simulink library "component_lib"  (R2020b)
settings: Solver=VariableStepAuto  StartTime=0.0  StopTime=10.0  RelTol=1e-3
undefined symbols (not defined in the file or in its folder): ECCV_r, par
libraries: base_lib x70, $bdroot x59, simulink x3, pid_lib x1
(part 1 of 3)
settings Model: Creator=maxjo65  LastModifiedBy=Max

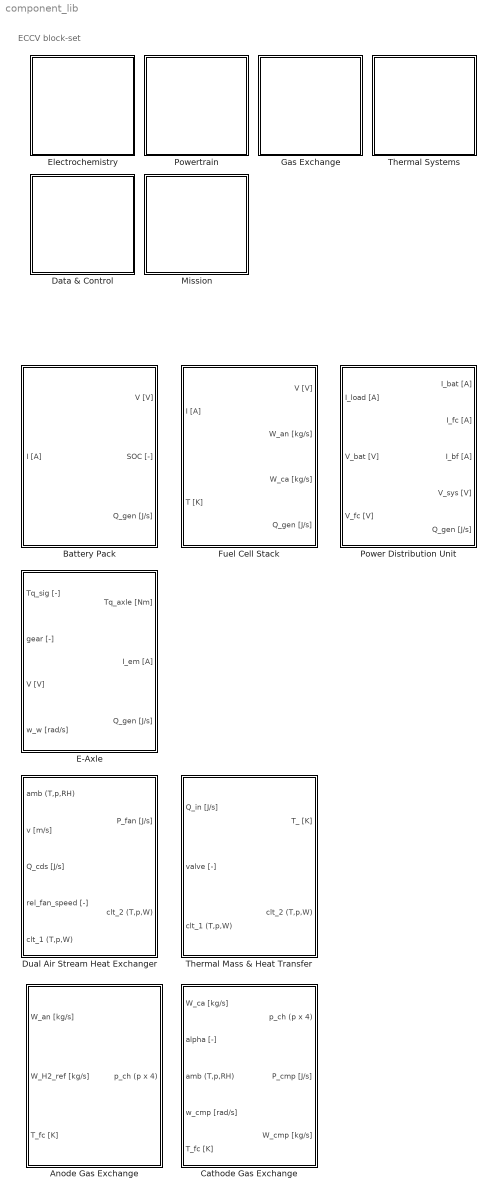
== system component_lib ==
  note: ECCV block-set
  Anode Gas Exchange : Subsystem
  Battery Pack : Subsystem  mask{SOC_0=0.5, Nx=74, Ny=6*16, T_bat=273 + 20}
      mask prompts: SOC_0 "Initial charge [-]:"; Nx "Cells in parallel  [-]:"; Ny "Cells in series [-]:"; T_bat "Temperature [K]:"
      mask init:
      | % parameter struct
      | par = struct;
      | 
      | % Get user-defined parameters
      | par.Ny = eval(get_param(gcb, 'Ny'));
      | par.Nx = eval(get_param(gcb, 'Nx'));
  Cathode Gas Exchange : Subsystem  mask{n_cell=335}
      mask prompts: n_cell "Nr. of cells [-]:"
  Data & Control : Subsystem
  Dual Air Stream Heat Exchanger : Subsystem  mask{HtH=1.1, StS=0.95}
      mask prompts: HtH "Header to header [m]"; StS "Sideplate to sideplate [m]"
  E-Axle : Subsystem  mask{n=2}
      mask prompts: n "Nr. of motors [-]"
  Electrochemistry : Subsystem
  Fuel Cell Stack : Subsystem  mask{N_series=335}
      mask prompts: N_series "Cells in series [#]:"
      mask init:
      | % parameter struct
      | par = struct;
      | 
      | % Get user-defined parameters
      | par.N_series   = eval(get_param(gcb, 'N_series'));
  Gas Exchange : Subsystem
  Mission : Subsystem
  Power Distribution Unit : Subsystem  mask{V_sys=420, P_fc=100e3, I_bt_max=300, I_bt_min=-150, T_s=1}
      mask prompts: V_sys "System voltage [V]:"; P_fc "Fuel cell power reference [J/s]:"; I_bt_max "Max. Battery current [A]"; I_bt_min "Min. Battery current [A]"; T_s "F.C Dynamic load time constant [s]:"
  Powertrain : Subsystem
  Thermal Mass & Heat Transfer : Subsystem  mask{n=5, d=2e-3, L=50e-2, m=150, cp=420, T_0=273 + 20}
      mask prompts: n "Channels [-]:"; d "Hydraulic diameter [m]:"; L "Length [m]:"; m "Mass [kg]:"; cp "Heat capacity [J/kgK]:"; T_0 "Initial temperature [K]:"
  Thermal Systems : Subsystem

== system component_lib/Anode Gas Exchange ==
  W_an [kg/s] : Inport
  W_H2_ref [kg/s] : Inport  Port=2
  T_fc [K] : Inport  Port=3
  Ejector : $bdroot/Gas Exchange/GE0013_simpleEjector  C_d=1  D_t=1.84e-3  Pi_lin=0.97  c_0=0.78406  c_1=-0.85801
  GE0007_hydrogenTank : $bdroot/Gas Exchange/GE0007_hydrogenTank  V=200e-3  T_tank=300  p_out=1.2e5  init_SOC=0.9  m0=5
  GE0008_gasProperties : $bdroot/Gas Exchange/GE0008_gasProperties  SystemSampleTime=-1  VariantActivationTime=update diagram  Latency=0  AutoFrameSizeCalculation=off
  Primary manifold : $bdroot/Gas Exchange/GE0009_controlVolume  V=10e-3  p0=5e5  x0_H2=1  x0_O2=0  T0=320  RH0=0
  SC0002_signalRead1 : $bdroot/Data & Control/SC0002_signalRead  SigName=anodeSupplyPartialPressure
  SC0002_signalRead2 : $bdroot/Data & Control/SC0002_signalRead  SigName=anodeSupplyPressure
  SC0002_signalRead3 : $bdroot/Data & Control/SC0002_signalRead  SigName=anodePrimaryPartialPressure
  SC0002_signalRead4 : $bdroot/Data & Control/SC0002_signalRead  SigName=entrainment
  SC0002_signalRead5 : $bdroot/Data & Control/SC0002_signalRead  SigName=recirculation
  SC0002_signalRead6 : $bdroot/Data & Control/SC0002_signalRead  SigName=anodePrimaryPressure
  SC0002_signalRead9 : $bdroot/Data & Control/SC0002_signalRead  SigName=anodeSupplyHumidity
  Sum1 : Sum  Inputs=++|
  Sum5 : Sum  Inputs=1
  Sum8 : Sum  Inputs=-+|
  Supply Manifold : $bdroot/Gas Exchange/GE0009_controlVolume  V=40e-3  p0=1.2e5  x0_H2=1  x0_O2=0  T0=320  RH0=0
  p_ch (p x 4) : Outport
  wires:
  Supply Manifold/2 -> GE0008_gasProperties/2
  GE0008_gasProperties/1 -> SC0002_signalRead2/1
  GE0008_gasProperties/2 -> SC0002_signalRead9/1
  Primary manifold/1 -> Ejector/1, Sum5/1, SC0002_signalRead3/1
  Sum5/1 -> SC0002_signalRead6/1
  W_H2_ref [kg/s]/1 -> GE0007_hydrogenTank/1
  GE0007_hydrogenTank/1 -> Sum8/2
  Sum8/1 -> Primary manifold/1
  GE0007_hydrogenTank/2 -> Primary manifold/2
  Primary manifold/2 -> Ejector/2
  Ejector/3 -> SC0002_signalRead5/1
  Ejector/4 -> SC0002_signalRead4/1
  Supply Manifold/1 -> Ejector/3, Ejector/5, GE0008_gasProperties/1, SC0002_signalRead1/1, p_ch (p x 4)/1
  T_fc [K]/1 -> Supply Manifold/2, Ejector/4
  Ejector/1 -> Sum1/2, Sum8/1
  Sum1/1 -> Supply Manifold/1
  W_an [kg/s]/1 -> Sum1/1

== system component_lib/Battery Pack ==
  I [A] : Inport
  Cell current : $bdroot/Data & Control/SC0002_signalRead  SigName=batteryCellCurrent
  Cell voltage : $bdroot/Data & Control/SC0002_signalRead  SigName=batteryCellVoltage
  Constant1 : Constant  Value=Nx
  Constant2 : Constant  Value=Ny
  Constant3 : Constant  Value=T_bat
  Constant4 : Constant  Value=Ny
  Constant5 : Constant  Value=Nx
  Divide : Product  Inputs=*/
  EL0001_panasonicNCR18650PF : $bdroot/Electrochemistry/EL0001_panasonicNCR18650PF  init_SOC=SOC_0
  Module current : $bdroot/Data & Control/SC0002_signalRead  SigName=batteryCurrent
  Module voltage : $bdroot/Data & Control/SC0002_signalRead  SigName=batteryVoltage
  Product1 : Product
  Product2 : Product  Inputs=3
  SOC : $bdroot/Data & Control/SC0002_signalRead  SigName=stateOfCharge
  battery power loss : $bdroot/Data & Control/SC0002_signalRead  SigName=batteryPowerLoss
  cell power loss : $bdroot/Data & Control/SC0002_signalRead  SigName=batteryCellPowerLoss
  V [V] : Outport
  SOC [-] : Outport  Port=2
  Q_gen [J/s] : Outport  Port=3
  wires:
  Product1/1 -> Module voltage/1, V [V]/1
  EL0001_panasonicNCR18650PF/2 -> SOC/1, SOC [-]/1
  Constant2/1 -> Product1/1
  EL0001_panasonicNCR18650PF/1 -> Cell voltage/1, Product1/2
  Divide/1 -> EL0001_panasonicNCR18650PF/1, Cell current/1
  I [A]/1 -> Module current/1, Divide/1
  Constant1/1 -> Divide/2
  Constant3/1 -> EL0001_panasonicNCR18650PF/2
  EL0001_panasonicNCR18650PF/3 -> Q_gen [J/s]/1, Product2/1, cell power loss/1
  Constant5/1 -> Product2/3
  Constant4/1 -> Product2/2
  Product2/1 -> battery power loss/1

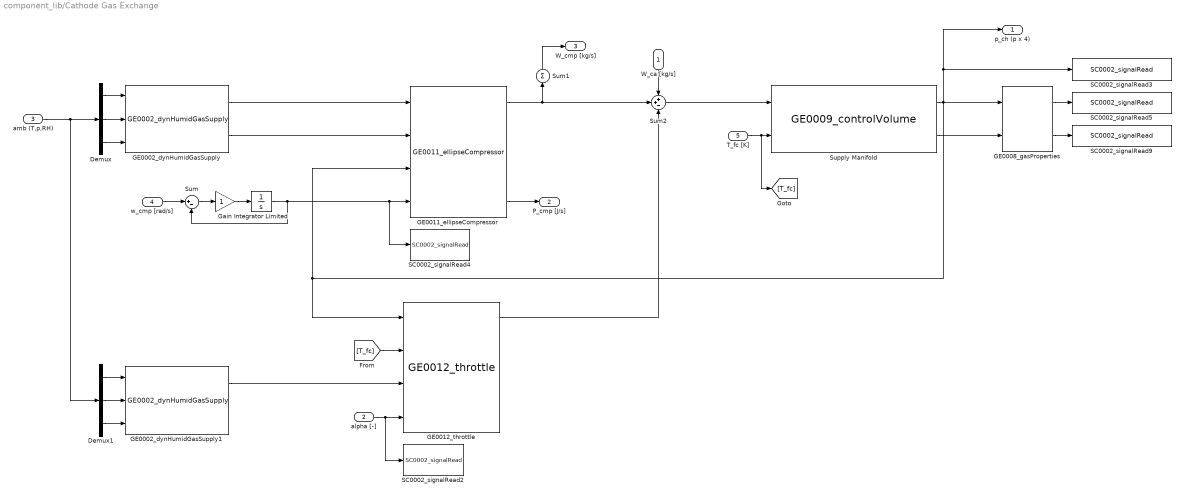
== system component_lib/Cathode Gas Exchange ==
  W_ca [kg/s] : Inport
  alpha [-] : Inport  Port=2
  amb (T,p,RH) : Inport  Port=3
  w_cmp [rad/s] : Inport  Port=4
  T_fc [K] : Inport  Port=5
  Demux : Demux  Outputs=3
  Demux1 : Demux  Outputs=3
  GE0002_dynHumidGasSupply : $bdroot/Gas Exchange/GE0002_dynHumidGasSupply  x_H2_dry=0  x_O2_dry=0.21
  GE0002_dynHumidGasSupply1 : $bdroot/Gas Exchange/GE0002_dynHumidGasSupply  x_H2_dry=0  x_O2_dry=0.21
  GE0008_gasProperties : $bdroot/Gas Exchange/GE0008_gasProperties  SystemSampleTime=-1  VariantActivationTime=update diagram  Latency=0  AutoFrameSizeCalculation=off
  GE0011_ellipseCompressor : $bdroot/Gas Exchange/GE0011_ellipseCompressor  w0=3e3
  GE0012_throttle : $bdroot/Gas Exchange/GE0012_throttle  a0=1.3229e-5  a1=9.4736e-5  a2=0.0029  Pi_lin=0.97  tan_par=1
  Gain : Gain
  Integrator Limited : Integrator  InitialCondition=1e4  LimitOutput=on  UpperSaturationLimit=2e4  LowerSaturationLimit=3e3
  SC0002_signalRead2 : $bdroot/Data & Control/SC0002_signalRead  SigName=throttlePosition
  SC0002_signalRead3 : $bdroot/Data & Control/SC0002_signalRead  SigName=cathodePartialPressure
  SC0002_signalRead4 : $bdroot/Data & Control/SC0002_signalRead  SigName=compressorSpeed
  SC0002_signalRead5 : $bdroot/Data & Control/SC0002_signalRead  SigName=cathodePressure
  SC0002_signalRead9 : $bdroot/Data & Control/SC0002_signalRead  SigName=cathodeHumidity
  Sum : Sum  Inputs=|+-
  Sum1 : Sum  Inputs=1
  Sum2 : Sum  Inputs=++-
  Supply Manifold : $bdroot/Gas Exchange/GE0009_controlVolume  V=20e-3  p0=2e5  x0_H2=0  x0_O2=0.21  T0=320  RH0=0
  p_ch (p x 4) : Outport
  P_cmp [J/s] : Outport  Port=2
  W_cmp [kg/s] : Outport  Port=3
  wires:
  GE0008_gasProperties/2 -> SC0002_signalRead9/1
  Supply Manifold/1 -> p_ch (p x 4)/1, SC0002_signalRead3/1, GE0008_gasProperties/1, GE0012_throttle/1, GE0011_ellipseCompressor/3
  GE0008_gasProperties/1 -> SC0002_signalRead5/1
  amb (T,p,RH)/1 -> Demux/1, Demux1/1
  Demux1/3 -> GE0002_dynHumidGasSupply1/3
  Demux1/2 -> GE0002_dynHumidGasSupply1/2
  Demux1/1 -> GE0002_dynHumidGasSupply1/1
  Demux/3 -> GE0002_dynHumidGasSupply/3
  Demux/2 -> GE0002_dynHumidGasSupply/2
  Demux/1 -> GE0002_dynHumidGasSupply/1
  alpha [-]/1 -> SC0002_signalRead2/1, GE0012_throttle/4
  GE0011_ellipseCompressor/4 -> P_cmp [J/s]/1
  Sum1/1 -> W_cmp [kg/s]/1
  Sum2/1 -> Supply Manifold/1
  GE0011_ellipseCompressor/1 -> Sum2/2, Sum1/1
  GE0002_dynHumidGasSupply/2 -> GE0011_ellipseCompressor/2
  T_fc [K]/1 -> [T_fc], Supply Manifold/2
  GE0002_dynHumidGasSupply1/1 -> GE0012_throttle/3
  GE0002_dynHumidGasSupply/1 -> GE0011_ellipseCompressor/1
  Supply Manifold/2 -> GE0008_gasProperties/2
  W_ca [kg/s]/1 -> Sum2/1
  GE0012_throttle/1 -> Sum2/3
  [T_fc] -> GE0012_throttle/2
  w_cmp [rad/s]/1 -> Sum/1
  Sum/1 -> Gain/1
  Integrator Limited/1 -> Sum/2, SC0002_signalRead4/1, GE0011_ellipseCompressor/4
  Gain/1 -> Integrator Limited/1

== system component_lib/Data & Control ==
  DC0006_powerSplit : Subsystem  mask{P_fc=100e3, P_fc_max=180e3, P_fc_min=10e3, T_s=1, I_bt_max=300, I_bt_min=-150}
      mask prompts: P_fc "FC power setpoint [J/s]:"; P_fc_max "Max. FC power [J/s]:"; P_fc_min "Min. FC power [J/s]:"; T_s "FC Dynamic load time constant [s]:"; I_bt_max "Max. battery current [A]:"; I_bt_min "Min. battery current [A]:"
  DC0007_cathodeFlowControl : Subsystem  mask{lambda_O2_ref=2, n_cell=455}
      mask prompts: lambda_O2_ref "Oxygen stoich. reference [-]:"; n_cell "Nr. of cells [-]:"
  DC0010_anodeTankFlowControl : Subsystem  mask{n_cell=455}
      mask prompts: n_cell "Nr. of cells [-]"
  SC0002_signalRead : Subsystem  mask{SigName=SigIdentifier}
      mask prompts: SigName "Signal identifier:"
      mask init:
      | % set name of input port
      | blockNames = Simulink.findBlocks(gcb);
      | set(blockNames(1), 'Name', SigName);
      | 
      | % log input port
      | ph = get_param([gcb, '/', SigName], 'PortHandles');
      | set_param(ph.Outport(1), 'DataLogging', 'on')
      | 
      | % set signal name in goto tag
      | set_param([gcb, '/', 'Goto'], 'GotoTag', SigName)
      mask Display: disp(SigName)
  SC0003_signalWrite : Subsystem  mask{SigName=SigIdentifier}
      mask prompts: SigName "Signal identifier:"
      mask init:
      | % set signal name in goto tag
      | set_param([gcb, '/', 'From'], 'GotoTag', SigName)
      mask Display: disp(SigName)

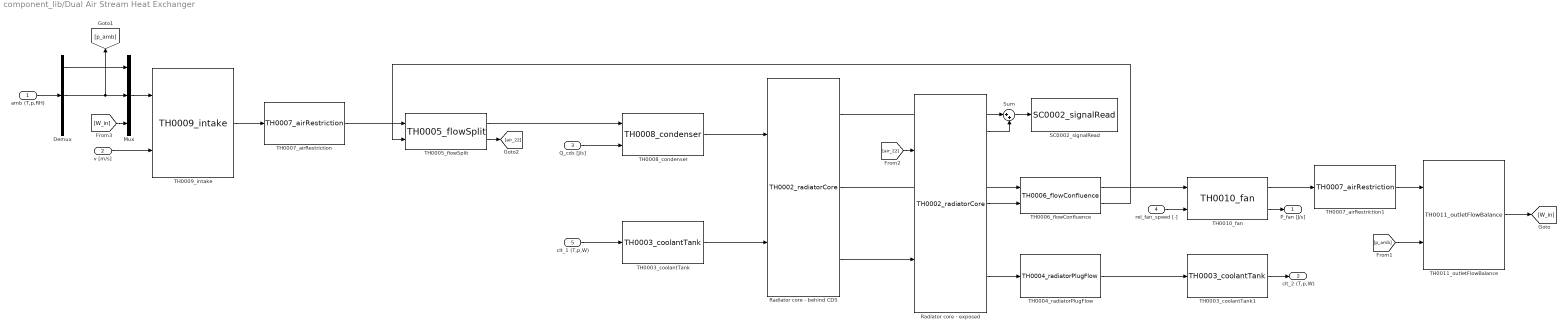
== system component_lib/Dual Air Stream Heat Exchanger ==
  amb (T,p,RH) : Inport
  v [m/s] : Inport  Port=2
  Q_cds [J/s] : Inport  Port=3
  rel_fan_speed [-] : Inport  Port=4
  clt_1 (T,p,W) : Inport  Port=5
  Demux : Demux  Outputs=3
  Mux : Mux  Inputs=3
  Radiator core - behind CDS : $bdroot/Thermal Systems/TH0002_radiatorCore  HtH=0.35  StS=0.95  radmodel=52 mm
  Radiator core - exposed : $bdroot/Thermal Systems/TH0002_radiatorCore  HtH=1.1-0.35  StS=0.95  radmodel=52 mm
  SC0002_signalRead : $bdroot/Data & Control/SC0002_signalRead  SigName=hexCoolingLoad
  Sum : Sum  Inputs=|++
  TH0003_coolantTank : $bdroot/Thermal Systems/TH0003_coolantTank  StS=0.95  D_con=0.055  T_0=286  radmodel=52 mm
  TH0003_coolantTank1 : $bdroot/Thermal Systems/TH0003_coolantTank  StS=0.95  D_con=0.055  T_0=286  radmodel=52 mm
  TH0004_radiatorPlugFlow : $bdroot/Thermal Systems/TH0004_radiatorPlugFlow  HtH=1.1  StS=0.95  T_0=286  radmodel=52 mm
  TH0005_flowSplit : $bdroot/Thermal Systems/TH0005_flowSplit  SystemSampleTime=-1  VariantActivationTime=update diagram  Latency=0  AutoFrameSizeCalculation=off
  TH0006_flowConfluence : $bdroot/Thermal Systems/TH0006_flowConfluence  gain=0.01
  TH0007_airRestriction : $bdroot/Thermal Systems/TH0007_airRestriction  A=0.8  zeta=0.3
  TH0007_airRestriction1 : $bdroot/Thermal Systems/TH0007_airRestriction  A=1  zeta=2.5
  TH0008_condenser : $bdroot/Thermal Systems/TH0008_condenser  HtH=0.85  StS=0.35  cdsmodel=18.8 mm
  TH0009_intake : $bdroot/Thermal Systems/TH0009_intake  zeta=0.9
  TH0010_fan : $bdroot/Thermal Systems/TH0010_fan  n_fan=4
  TH0011_outletFlowBalance : $bdroot/Thermal Systems/TH0011_outletFlowBalance  gain=0.05
  P_fan [J/s] : Outport
  clt_2 (T,p,W) : Outport  Port=2
  wires:
  Demux/2 -> Mux/2, [p_amb]
  Demux/1 -> Mux/1
  amb (T,p,RH)/1 -> Demux/1
  TH0003_coolantTank1/1 -> clt_2 (T,p,W)/1
  Sum/1 -> SC0002_signalRead/1
  TH0010_fan/2 -> P_fan [J/s]/1
  rel_fan_speed [-]/1 -> TH0010_fan/2
  TH0005_flowSplit/1 -> TH0008_condenser/1
  Radiator core - behind CDS/1 -> Sum/1
  v [m/s]/1 -> TH0009_intake/2
  TH0007_airRestriction/1 -> TH0005_flowSplit/1
  TH0004_radiatorPlugFlow/1 -> TH0003_coolantTank1/1
  TH0007_airRestriction1/1 -> TH0011_outletFlowBalance/1
  TH0003_coolantTank/1 -> Radiator core - behind CDS/2
  Q_cds [J/s]/1 -> TH0008_condenser/2
  clt_1 (T,p,W)/1 -> TH0003_coolantTank/1
  TH0006_flowConfluence/2 -> TH0005_flowSplit/2
  TH0006_flowConfluence/1 -> TH0010_fan/1
  Mux/1 -> TH0009_intake/1
  TH0005_flowSplit/2 -> [air_22]
  TH0009_intake/1 -> TH0007_airRestriction/1
  TH0008_condenser/1 -> Radiator core - behind CDS/1
  Radiator core - behind CDS/2 -> TH0006_flowConfluence/1
  Radiator core - exposed/2 -> TH0006_flowConfluence/2
  Radiator core - behind CDS/3 -> Radiator core - exposed/2
  [p_amb] -> TH0011_outletFlowBalance/2
  [air_22] -> Radiator core - exposed/1
  TH0010_fan/1 -> TH0007_airRestriction1/1
  Radiator core - exposed/3 -> TH0004_radiatorPlugFlow/1
  TH0011_outletFlowBalance/1 -> [W_in]
  Radiator core - exposed/1 -> Sum/2
  [W_in] -> Mux/3

== system component_lib/E-Axle ==
  note: Input as % of max. torque at current speed
  Tq_sig [-] : Inport
  gear [-] : Inport  Port=2
  V [V] : Inport  Port=3
  w_w [rad/s] : Inport  Port=4
  Constant3 : Constant
  Current sensor : $bdroot/Data & Control/SC0002_signalRead  SigName=motorCurrent
  Divide3 : Product  Inputs=**
  Gain : Gain  Gain=n
  Gain1 : Gain  Gain=n
  Gain2 : Gain  Gain=n
  Max torque : $bdroot/Data & Control/SC0002_signalRead  SigName=maxMotorTorque
  PT0002_simpleMotor : $bdroot/Powertrain/PT0002_simpleMotor  T_s=0.1
  PT0003_gearBox : $bdroot/Powertrain/PT0003_gearBox  fd_ratio=5  gear_ratios=[1, 1]  eta_gb=0.98
  Saturation : Saturate  UpperLimit=1  LowerLimit=-1
  Saturation1 : Saturate  UpperLimit=476  LowerLimit=0
  Speed sensor : $bdroot/Data & Control/SC0002_signalRead  SigName=motorSpeed
  Torque sensor : $bdroot/Data & Control/SC0002_signalRead  SigName=motorTorque
  speed-Torque map : Lookup_n-D  NumberOfTableDimensions=1  BreakpointsForDimension1=|  Table=|  InternalRulePriority=Speed  RndMeth=Simplest  InputSameDT=on
      BreakpointsForDimension1=|
      | [25.2590673575129
      | 34.9740932642487
      | 43.3937823834197
      | 51.1658031088083
      | 55.6994818652850
      | 64.1191709844560
      | 65.4145077720207
      | 67.3575129533679
      | 68.0051813471503
      | 69.9481865284974
      | 71.2435233160622
      | 73.1865284974093
      | 75.7772020725389
      | 76.4248704663213
      | 78.3678756476684
      | 81.6062176165803
      | 82.9015544041451
      | 86.1398963730570
      | 88.0829015544041
      | 90.0259067357513
      | 94.5595854922280
      | 97.1502590673575
      | 100.388601036269
      | 103.626943005181
      | 109.455958549223
      | 113.989637305699
      | 120.466321243523
      | 125.000000000000
      | 128.238341968912
      | 133.419689119171
      | 139.248704663212
      | 145.077720207254
      | 150.259067357513
      | 158.031088082902
      | 164.507772020725
      | 172.279792746114
      | 174.870466321244
      | 195.595854922280
      | 211.139896373057
      | 221.502590673575
      | 229.922279792746
      | 244.818652849741
      | 256.476683937824
      | 270.725388601036
      | 284.974093264249
      | 290.155440414508
      | 300.518134715026
      | 313.471502590674
      | 324.481865284974
      | 344.559585492228
      | 356.217616580311
      | 366.580310880829
      | 376.295336787565
      | 384.067357512953
      | 403.497409326425
      | 422.927461139896
      | 438.471502590674
      | 453.367875647669
      | 465.025906735751
      | 476.036269430052]
      Table=|
      | [1991.26637554585
      | 1997.08879184862
      | 1994.17758369723
      | 1994.17758369723
      | 1994.17758369723
      | 1991.26637554585
      | 1944.68704512373
      | 1921.39737991266
      | 1854.43959243086
      | 1816.59388646288
      | 1787.48180494905
      | 1700.14556040757
      | 1671.03347889374
      | 1621.54294032023
      | 1548.76273653566
      | 1513.82823871907
      | 1438.13682678311
      | 1391.55749636099
      | 1339.15574963610
      | 1280.93158660844
      | 1225.61863173217
      | 1176.12809315866
      | 1129.54876273654
      | 1085.88064046579
      | 1018.92285298399
      | 969.432314410480
      | 925.764192139738
      | 876.273653566230
      | 835.516739446870
      | 797.671033478894
      | 756.914119359534
      | 727.802037845706
      | 704.512372634643
      | 666.666666666667
      | 628.820960698690
      | 602.620087336244
      | 588.064046579330
      | 518.195050946142
      | 477.438136826783
      | 445.414847161572
      | 410.480349344978
      | 395.924308588064
      | 375.545851528384
      | 343.522561863173
      | 328.966521106259
      | 320.232896652110
      | 302.765647743814
      | 282.387190684134
      | 282.387190684134
      | 259.097525473071
      | 244.541484716157
      | 244.541484716157
      | 221.251819505094
      | 221.251819505094
      | 209.606986899563
      | 195.050946142649
      | 189.228529839883
      | 183.406113537118
      | 174.672489082969
      | 157.205240174672]
  Tq_axle [Nm] : Outport
  I_em [A] : Outport  Port=2
  Q_gen [J/s] : Outport  Port=3
  wires:
  Gain2/1 -> Tq_axle [Nm]/1
  PT0003_gearBox/1 -> Gain2/1
  PT0002_simpleMotor/3 -> Gain/1
  Gain1/1 -> I_em [A]/1
  PT0002_simpleMotor/1 -> Torque sensor/1, PT0003_gearBox/1
  Divide3/1 -> PT0002_simpleMotor/1
  Constant3/1 -> PT0003_gearBox/4
  gear [-]/1 -> PT0003_gearBox/3
  Tq_sig [-]/1 -> Saturation/1
  Saturation1/1 -> speed-Torque map/1
  PT0003_gearBox/2 -> Saturation1/1, PT0002_simpleMotor/3, Speed sensor/1
  w_w [rad/s]/1 -> PT0003_gearBox/2
  Saturation/1 -> Divide3/1
  speed-Torque map/1 -> Max torque/1, Divide3/2
  PT0002_simpleMotor/2 -> Current sensor/1, Gain1/1
  V [V]/1 -> PT0002_simpleMotor/2
  Gain/1 -> Q_gen [J/s]/1

== system component_lib/Electrochemistry ==
  EL0001_panasonicNCR18650PF : Subsystem  mask{init_SOC=0.2380}
      mask prompts: init_SOC "Initial SOC [-]:"
      mask init:
      | % parameter struct
      | par = struct;
      | 
      | % Get user-defined parameters
      | par.init_SOC   = init_SOC;
  EL0003_pCell : Subsystem  mask{U_0=1, j_0=1e-3, alpha=0.25, ASR=1e-1, A_fc=300}
      mask prompts: U_0 "Open circuit voltage [V]:"; j_0 "Exchange current density [A/cm2]:"; alpha "Act. bar. symmetry [-]:"; ASR "Area specific resistance [ohm*cm2]:"; A_fc "Membrane area [cm2]:"
      mask init:
      | % parameter struct
      | par = struct;
      | 
      | % Get user-defined parameters
      | par.j_0   = j_0;
      | par.alpha = alpha;
      | par.ASR   = ASR;
      | par.U_0   = U_0;
      | par.A_fc  = A_fc;
      | 
      | % membrane thickness
      | par.t_m    = 0.01275;
      | 
      | % Molar mass - [kg/mol]
      | par.M_j  = [0.002;
      |             0.032;
      |             0.018;
      |             0.028];    
      | 
      | % Specific heat - [J/kg*K]        
      | par.cp_j = [14.43e3;
      |             0.928e3;
      |             1.996e3;
      |             1.041e3];  
      | 
      | % Universal gas constant - [J/(mol*K)]   
      | par.R  = 8.314;         
      | 
      | % Specific gas constant [J/kg*K]
      | par.R_j = par.R ./ par.M_j;
  EL0004_buckCCM : Subsystem  mask{C=1, L=1, eta=0.9, V_init=400}
      mask prompts: C "Capacity [F]:"; L "Inductance [H]:"; eta "Efficiency [-]:"; V_init "Voltage initial condition [V]:"
  EL0005_boostCCM : Subsystem  mask{C=1, L=1, eta=0.9, V_init=420}
      mask prompts: C "Capacity [F]:"; L "Inductance [H]:"; eta "Efficiency [-]:"; V_init "Voltage initial condition [V]:"
  EL0006_parallelVoltageSources : Subsystem  mask{R=1e-2, C=1, V_init=420}
      mask prompts: R "Resistance [Ohm]:"; C "Capacitance [F]:"; V_init "Voltage initial condition [V]:"

== system component_lib/Fuel Cell Stack ==
  I [A] : Inport
  T [K] : Inport  Port=2
  Constant4 : Constant  Value=par.N_series
  EL0003_pCell : $bdroot/Electrochemistry/EL0003_pCell  U_0=1  j_0=1e-3  alpha=0.25  ASR=1e-1  A_fc=300
  Product{1..3,5} (4 alike) : Product
  V [V] : Outport
  W_an [kg/s] : Outport  Port=2
  W_ca [kg/s] : Outport  Port=3
  Q_gen [J/s] : Outport  Port=4
  wires:
  Product1/1 -> V [V]/1
  EL0003_pCell/1 -> Product1/1
  Product2/1 -> W_an [kg/s]/1
  Product5/1 -> W_ca [kg/s]/1
  Constant4/1 -> Product5/2, Product2/2, Product3/2, Product1/2
  I [A]/1 -> EL0003_pCell/1
  EL0003_pCell/4 -> Product5/1
  EL0003_pCell/3 -> Product2/1
  EL0003_pCell/2 -> Product3/1
  Product3/1 -> Q_gen [J/s]/1
  T [K]/1 -> EL0003_pCell/2

== system component_lib/Gas Exchange ==
  GE0001_humidGasSupply : Subsystem  mask{p_tot=1.01e5, x_H2=0, x_O2=0.21, RH=0, T=300}
      mask prompts: p_tot "Pressure [Pa]:"; x_H2 "Mole fraction dry H2 [-]:"; x_O2 "Mole fraction dry O2 [-]:"; RH "Relative humidity [-]:"; T "Temperature [K]:"
      mask init:
      | % parameter struct
      | par = struct;
      | 
      | par.p_tot = p_tot;
      | par.x_H2  = x_H2;
      | par.x_O2  = x_O2;
      | par.RH    = RH;
      | par.T     = T;
      | 
      | % par.p_tot = eval(get_param(gcb, 'p_tot'));
      | % par.x_H2  = eval(get_param(gcb, 'x_H2'));
      | % par.x_O2  = eval(get_param(gcb, 'x_O2'));
      | % par.RH    = eval(get_param(gcb, 'RH'));
      | % par.T     = eval(get_param(gcb, 'T'));
      | 
      | 
      | 
      | % Fixed parameters
      | par.R     = 8.314;  % [J/(mol*K)] - universal gas constant
      | par.M_N2  = 0.028;  % [kg/mol] - nitrogen molecular weight
      | par.M_H2O = 0.018;  % [kg/mol] - water
  GE0002_dynHumidGasSupply : Subsystem  mask{x_H2_dry=0, x_O2_dry=0.21}
      mask prompts: x_H2_dry "Mole-fraction dry hydrogen [-]:"; x_O2_dry "Mole-fraction dry oxygen [-]:"
      mask init:
      | % parameter struct
      | par = struct;
      | 
      | % Fixed parameters
      | par.R     = 8.314; % [J/(mol*K)] - universal gas constant
      | par.M_N2  = 0.028; % [kg/mol] - nitrogen molecular weight
      | par.M_H2O = 0.018; % [kg/mol] - water
  GE0007_hydrogenTank : Subsystem  mask{V=200e-3, T_tank=300, p_out=1.2e5, init_SOC=0.9, m0=5}
      mask prompts: V "Volume [m3]:"; T_tank "Tank temperature [K]:"; p_out "Outlet pressure [Pa]"; init_SOC "Initial charge [-]"; m0 "Total capacity [kg]:"
      mask init:
      | % parameter struct
      | par = struct;
      | 
      | % Get user-specified parameters
      | % par.V        = eval(get_param(gcb, 'V'));
      | % par.T_tank   = eval(get_param(gcb, 'T_tank'));
      | % par.p_out    = eval(get_param(gcb, 'p_out'));
      | % par.init_SOC = eval(get_param(gcb, 'init_SOC'));
      | % par.m0       = eval(get_param(gcb, 'm0'));
      | 
      | par.V        = V;
      | par.T_tank   = T_tank;
      | par.p_out    = p_out;
      | par.init_SOC = init_SOC;
      | par.m0       = m0;
      | 
      | 
      | % Standard state values
      | par.T0 = 298.15;  % [K]     - standard state temperature
      | par.h0 = 7.9260e3; % [J/mol] - standard state enthalpy
      | 
      | % Molar mass - [kg/mol]
      | par.M_j  = [0.002;
      |             0.032;
      |             0.018;
      |             0.028];    
      | 
      | % Specific heat - [J/kg*K]        
      | par.cp_j = [14.43e3;
      |             0.928e3;
      |             1.996e3;
      |             1.041e3];  
      | 
      | % Universal gas constant - [J/(mol*K)]   
      | par.R  = 8.314;         
      | 
      | % Specific gas constant [J/kg*K]
      | par.R_j = par.R ./ par.M_j;
  GE0008_gasProperties : Subsystem
  GE0009_controlVolume : Subsystem  mask{V=1.5833e-05, p0=1.01e5, x0_H2=0, x0_O2=0.21, T0=320, RH0=0}
      mask prompts: V "Volume [m3]:"; p0 "Pressure [Pa]:"; x0_H2 "Mole fraction dry H2 [-]:"; x0_O2 "Mole fraction dry O2 [-]:"; T0 "Temperature [K]:"; RH0 "Relative humidity [-]:"
      mask init:
      | % parameter struct
      | par = struct;
      | 
      | % Get user-specified parameters
      | % par.V   = eval(get_param(gcb, 'V'));
      | par.V = V;
      | 
      | % initial conditions
      | par.p0    = p0;
      | par.x0_H2 = x0_H2;
      | par.x0_O2 = x0_O2;
      | par.T0    = T0;
      | par.RH0   = RH0;
      | 
      | % par.p0    = eval(get_param(gcb, 'p0'));
      | % par.x0_H2 = eval(get_param(gcb, 'x0_H2'));
      | % par.x0_O2 = eval(get_param(gcb, 'x0_O2'));
      | % par.T0    = eval(get_param(gcb, 'T0'));
      | % par.RH0   = eval(get_param(gcb, 'RH0'));
      | 
      | % Molar mass - [kg/mol]
      | par.M_j  = [0.002;
      |             0.032;
      |             0.018;
      |             0.028];    
      | 
      | % Specific heat - [J/kg*K]        
      | par.cp_j = [14.43e3;
      |             0.928e3;
      |             1.996e3;
      |             1.041e3];  
      | 
      | % Universal gas constant - [J/(mol*K)]   
      | par.R  = 8.314;         
      | 
      | % Specific gas constant [J/kg*K]
      | par.R_j = par.R ./ par.M_j;
      mask DialogControl Container3 Prompt: Initial conditions:
  GE0010_flowRestriction : Subsystem  mask{C_d=1, D_t=1.84e-3, Pi_lin=0.97, tan_par=1}
      mask prompts: C_d "Discharge coefficient [-]:"; D_t "Throat diameter [m]:"; Pi_lin "Lin. region  [-]"; tan_par "Tanhyp parameter [-]:"
      mask init:
      | % Check side
      | par = struct;
      | 
      | % parameters
      | % par.C_d     = eval(get_param(gcb, 'C_d'));
      | % par.Pi_lin  = eval(get_param(gcb, 'Pi_lin'));
      | % par.D_t     = eval(get_param(gcb, 'D_t'));
      | % par.tan_par = eval(get_param(gcb, 'tan_par'));
      | 
      | par.C_d     = C_d;
      | par.Pi_lin  = Pi_lin;
      | par.D_t     = D_t;
      | par.tan_par = tan_par;
      | 
      | % Molar mass - [kg/mol]
      | par.M_j  = [0.002;
      |             0.032;
      |             0.018;
      |             0.028];    
      | 
      | % Specific heat - [J/kg*K]        
      | par.cp_j = [14.43e3;
      |             0.928e3;
      |             1.996e3;
      |             1.041e3];  
      | 
      | % Universal gas constant - [J/(mol*K)]   
      | par.R  = 8.314;         
      | 
      | % Specific gas constant [J/kg*K]
      | par.R_j = par.R ./ par.M_j;
  GE0011_ellipseCompressor : Subsystem  mask{w0=3e3}
      mask prompts: w0 "Initial speed [rad/s]:"
      mask init:
      | % parameter struct
      | par = struct;
      | 
      | % Get user-specified parameters
      | % par.w0   = eval(get_param(gcb, 'w0'));
      | par.w0   = w0;
      | 
      | % Compressor parameters
      | par.C_Wch       = [0.791459084209095;0.278369840595707;2.56393896117876;1.42688664691882];
      | par.C_PIch      = [0.0903657853262553;0.467638667413134;4.35616456423884]; 
      | par.C_Wzs       = [0.851951915665070;2.98625689994966];
      | par.C_PIzs      = [1.24697676678299;2.08506798865712];
      | par.C_cur       = [2.08068646432419;4.30416619749832;5.84893356036723];
      | par.Gamma_PIcs  = [0.500000000000000];
      | par.C_s         = [1.47023010236244];
      | par.C_b         = [1.806586538255675;-0.642454577867690];
      | par.C_a         = [0.863755184943499;0.033339263835893;24.999999984802365];
      | par.C_loss      = 0.009455201151738;
      | par.T_ref       =  298;
      | par.p_ref       = 100000;
      | par.Nc_max_map  = 1.860592187500000e+05;
      | par.Wc_max_map  = 0.252151000000000;
      | par.PI_max_map  = 2.766539113153419;
      | par.Delta_h_max = 1.738661132271557e+05;
      | par.gamma_air   = 1.397693997445722;
      | par.rho1        = 1.169072149521521;
      | par.D_2         = 0.056300000000000;
      | par.Cp_air      = 1.008800956523303e+03;
      | par.alpha_kPiW0 = 1.645763320284325;
      | par.J_c         = 1.730000000000000e-05;
      | par.c_fric      = 1e-6;
      | 
      | 
      | % Molar mass - [kg/mol]
      | par.M_j  = [0.002;
      |             0.032;
      |             0.018;
      |             0.028];    
      | 
      | % Specific heat - [J/kg*K]        
      | par.cp_j = [14.43e3;
      |             0.928e3;
      |             1.996e3;
      |             1.041e3];  
      | 
      | % Universal gas constant - [J/(mol*K)]   
      | par.R  = 8.314;         
      | 
      | % Specific gas constant [J/kg*K]
      | par.R_j = par.R ./ par.M_j;
  GE0012_throttle : Subsystem  mask{a0=1.3229e-5, a1=9.4736e-5, a2=0.0029, Pi_lin=0.97, tan_par=1}
      mask prompts: Pi_lin "Lin. region [-]:"; tan_par "Tanhyp parameter [-]:"
      mask init:
      | % parameter struct
      | par = struct;
      | 
      | % Get user-specified parameters
      | % par.a0      = eval(get_param(gcb, 'a0'));
      | % par.a1      = eval(get_param(gcb, 'a1'));
      | % par.a2      = eval(get_param(gcb, 'a2'));
      | % par.Pi_lin  = eval(get_param(gcb, 'Pi_lin'));
      | % par.tan_par = eval(get_param(gcb, 'tan_par'));
      | 
      | par.a0      = a0;
      | par.a1      = a1;
      | par.a2      = a2;
      | par.Pi_lin  = Pi_lin;
      | par.tan_par = tan_par;
      | 
      | 
      | % Molar mass - [kg/mol]
      | par.M_j  = [0.002;
      |             0.032;
      |             0.018;
      |             0.028];    
      | 
      | % Specific heat - [J/kg*K]        
      | par.cp_j = [14.43e3;
      |             0.928e3;
      |             1.996e3;
      |             1.041e3];  
      | 
      | % Universal gas constant - [J/(mol*K)]   
      | par.R  = 8.314;         
      | 
      | % Specific gas constant [J/kg*K]
      | par.R_j = par.R ./ par.M_j;
  GE0013_simpleEjector : Subsystem  mask{C_d=1, D_t=1.84e-3, Pi_lin=0.97, c_0=0.78406, c_1=-0.85801}
      mask prompts: C_d "Discharge coefficient [-]:"; D_t "Nozzle throat diameter [m]:"; Pi_lin "Linear region [-]:"; c_0 "c0"; c_1 "c1"
      mask init:
      | % parameter struct
      | par = struct;
      | 
      | % Get user-specified parameters
      | % par.C_d    = eval(get_param(gcb, 'C_d'));
      | % par.D_t    = eval(get_param(gcb, 'D_t'));
      | % par.Pi_lin = eval(get_param(gcb, 'Pi_lin'));
      | % par.c_0     = eval(get_param(gcb, 'c_0'));
      | % par.c_1     = eval(get_param(gcb, 'c_1'));
      | 
      | par.C_d    = C_d;
      | par.D_t    = D_t;
      | par.Pi_lin = Pi_lin;
      | par.c_0    = c_0;
      | par.c_1    = c_1;
      |  
      | % Molar mass - [kg/mol]
      | par.M_j  = [0.002;
      |             0.032;
      |             0.018;
      |             0.028];    
      | 
      | % Specific heat - [J/kg*K]        
      | par.cp_j = [14.43e3;
      |             0.928e3;
      |             1.996e3;
      |             1.041e3];  
      | 
      | % Universal gas constant - [J/(mol*K)]   
      | par.R  = 8.314;         
      | 
      | % Specific gas constant [J/kg*K]
      | par.R_j = par.R ./ par.M_j;
  GE0014_flowValve : Subsystem  mask{C_d=1, D_t=1.84e-3, Pi_lin=0.97, tan_par=1}
      mask prompts: C_d "Discharge coefficient [-]:"; D_t "Throat diameter [m]:"; Pi_lin "Lin. region  [-]"; tan_par "Tanhyp parameter [-]:"
      mask init:
      | % Check side
      | par = struct;
      | 
      | % parameters
      | % par.C_d     = eval(get_param(gcb, 'C_d'));
      | % par.Pi_lin  = eval(get_param(gcb, 'Pi_lin'));
      | % par.D_t     = eval(get_param(gcb, 'D_t'));
      | % par.tan_par = eval(get_param(gcb, 'tan_par'));
      | 
      | par.C_d     = C_d;
      | par.Pi_lin  = Pi_lin;
      | par.D_t     = D_t;
      | par.tan_par = tan_par;
      | 
      | 
      | % Molar mass - [kg/mol]
      | par.M_j  = [0.002;
      |             0.032;
      |             0.018;
      |             0.028];    
      | 
      | % Specific heat - [J/kg*K]        
      | par.cp_j = [14.43e3;
      |             0.928e3;
      |             1.996e3;
      |             1.041e3];  
      | 
      | % Universal gas constant - [J/(mol*K)]   
      | par.R  = 8.314;         
      | 
      | % Specific gas constant [J/kg*K]
      | par.R_j = par.R ./ par.M_j;
  GE0015_linearRestriction : Subsystem  mask{C_d=4.7083e-08, tan_par=1}
      mask prompts: C_d "Discharge coefficient [-]:"; tan_par "Tanhyp parameter [-]:"
      mask init:
      | % Check side
      | par = struct;
      | 
      | % parameters
      | % par.C_d     = eval(get_param(gcb, 'C_d'));
      | % par.tan_par = eval(get_param(gcb, 'tan_par'));
      | 
      | par.C_d     = C_d;
      | par.tan_par = tan_par;
      | 
      | % Molar mass - [kg/mol]
      | par.M_j  = [0.002;
      |             0.032;
      |             0.018;
      |             0.028];    
      | 
      | % Specific heat - [J/kg*K]        
      | par.cp_j = [14.43e3;
      |             0.928e3;
      |             1.996e3;
      |             1.041e3];  
      | 
      | % Universal gas constant - [J/(mol*K)]   
      | par.R  = 8.314;         
      | 
      | % Specific gas constant [J/kg*K]
      | par.R_j = par.R ./ par.M_j;

== system component_lib/Mission ==
  MN0001_profile : Subsystem  mask{profile=KoblenzTrier.mat, x0=0, N_lookahead=100}
      mask prompts: profile "Road profile:"; x0 "Starting distance [m]:"; N_lookahead "Lookahead horizon [-]:"
      mask init:
      | % find road profiles in folder
      | availableProfiles = dir(fullfile('road_profiles','*.mat'));
      | availableProfiles = {availableProfiles.name};
      | 
      | % update popup_list
      | msk = Simulink.Mask.get(gcb);
      | msk.Parameters(1).TypeOptions = availableProfiles;
      | 
      | % set profile
      | try
      |     load(profile);
      | end
      mask TypeOptions profile: KoblenzTrier.mat | Munchen.mat | Sodertalje_Norrkoping.mat
      mask Display:
      | try
      |     plot(ECCV_r.distance, ECCV_r.altitude)
      | end
  MN0002_ambient : Subsystem  mask{p_0=1.01e5, T_0=298, RH_0=0.2}
      mask prompts: p_0 "Sea-level pressure [Pa]:"; T_0 "Sea-level temperature [K]:"; RH_0 "Sea-level humidity [-]:"
      mask init:
      | % parameter struct
      | par = struct;
      | 
      | % initial conditions
      | % par.p_0 = eval(get_param(gcb, 'p_0'));
      | % par.T_0 = eval(get_param(gcb, 'T_0'));
      | 
      | par.p_0 = p_0;
      | par.T_0 = T_0;

== system component_lib/Power Distribution Unit ==
  note: Filter to avoid algebraic loop
  note: Filter to avoid algebraic loop
  I_load [A] : Inport
  V_bat [V] : Inport  Port=2
  V_fc [V] : Inport  Port=3
  Abs : Abs
  Constant : Constant  Value=V_sys
  DC0006_powerSplit : $bdroot/Data & Control/DC0006_powerSplit  P_fc=P_fc  P_fc_max=180e3  P_fc_min=10e3  T_s=T_s  I_bt_max=I_bt_max  I_bt_min=I_bt_min
  Gain1 : Gain  Gain=1e3
  Gain2 : Gain  Gain=1e3
  Integrator : Integrator  InitialCondition=600
  Integrator1 : Integrator  InitialCondition=300
  Product : Product
  Product1 : Product
  SC0002_signalRead1 : $bdroot/Data & Control/SC0002_signalRead  SigName=requiredPower
  SC0002_signalRead7 : $bdroot/Data & Control/SC0002_signalRead  SigName=burnOffPower
  Sum : Sum  Inputs=|+-
  Sum1 : Sum  Inputs=|+-
  I_bat [A] : Outport
  I_fc [A] : Outport  Port=2
  I_bf [A] : Outport  Port=3
  V_sys [V] : Outport  Port=4
  Q_gen [J/s] : Outport  Port=5
  wires:
  Product1/1 -> SC0002_signalRead7/1, Abs/1
  DC0006_powerSplit/1 -> I_bat [A]/1
  DC0006_powerSplit/2 -> I_fc [A]/1
  Constant/1 -> DC0006_powerSplit/4, Product1/2, Product/2, V_sys [V]/1
  I_load [A]/1 -> Product/1
  Product/1 -> DC0006_powerSplit/1, SC0002_signalRead1/1
  Sum1/1 -> Gain2/1
  Gain2/1 -> Integrator1/1
  V_fc [V]/1 -> Sum1/1
  Integrator1/1 -> DC0006_powerSplit/2, Sum1/2
  Gain1/1 -> Integrator/1
  V_bat [V]/1 -> Sum/1
  Integrator/1 -> Sum/2, DC0006_powerSplit/3
  Sum/1 -> Gain1/1
  DC0006_powerSplit/3 -> Product1/1, I_bf [A]/1
  Abs/1 -> Q_gen [J/s]/1

== system component_lib/Powertrain ==
  PT0001_simpleVehicle : Subsystem  mask{m=10e3, r_w=0.5, A_f=10, C_d=0.5, rho_air=1.225, c_r0=0.0060, c_r1=2.3e-7, gain=600, v0=0, x0=0}
      mask prompts: m "Vehicle mass [kg]:"; r_w "Wheel radius [m]:"; A_f "area [m2]:"; C_d "Flow coefficient:"; rho_air "air density [kg/m3]:"; v0 "Initial speed [m/s]:"; x0 "Initial position [m]:"
      mask init:
      | % parameter struct
      | par = struct;
      | 
      | % Get user-defined parameters
      | par.m        = m;
      | par.r_w      = r_w;
      | par.A_f      = A_f;
      | par.C_d      = C_d;
      | par.rho_air  = rho_air;
      | par.c_r0     = c_r0;
      | par.c_r1     = c_r1;
      | par.gain     = gain;
      | par.v0       = v0;
      | par.x0       = x0;
      mask DialogControl ParameterGroupVar Prompt: General
      mask DialogControl Container5 Prompt: Air drag
      mask DialogControl Container4 Prompt: Rolling resistance
      mask DialogControl Container7 Prompt: Brake
      mask DialogControl Container3 Prompt: Initial conditions
  PT0002_simpleMotor : Subsystem  mask{T_s=0.1}
      mask prompts: T_s "Torque time cont. [s]:"
      mask init:
      | % parameter struct
      | par = struct;
      | 
      | % motor parameters
      | par.e  = 1.2215;
      | par.c1 = 905.3796;
      | par.c2 = -53.7358;
      | par.c3 = 0.1681;
  PT0003_gearBox : Subsystem  mask{fd_ratio=5, gear_ratios=[1 2.59], eta_gb=0.98}
      mask prompts: fd_ratio "Final drive ratio [-]:"; gear_ratios "Gear ratios [-]:"; eta_gb "Efficiency [-]:"
      mask init:
      | % parameters
      | par = struct;
      | 
      | par.fd_ratio    = fd_ratio;
      | par.gear_ratios = gear_ratios;
      | par.eta_gb      = eta_gb;
      | par.gears       = 1:length(par.gear_ratios);

== system component_lib/Thermal Mass & Heat Transfer ==
  Q_in [J/s] : Inport
  valve [-] : Inport  Port=2
  clt_1 (T,p,W) : Inport  Port=3
  Gain3 : Gain  Gain=n
  Sum : Sum  Inputs=|+-
  TH0011_coolingChannel : $bdroot/Thermal Systems/TH0011_coolingChannel  d=10e-3  L=30e-2  n_ch=100
  TH0011_thermalMass : $bdroot/Thermal Systems/TH0011_thermalMass  m=m  cp=cp  T_0=T_0
  bypass valve : $bdroot/Thermal Systems/TH0014_valve  d=10e-2  dr=5e-2  C_d=0.9
  flow merge : $bdroot/Thermal Systems/TH0006_flowConfluence  gain=1e-4
  T_ [K] : Outport
  clt_2 (T,p,W) : Outport  Port=2
  wires:
  flow merge/1 -> clt_2 (T,p,W)/1
  TH0011_coolingChannel/2 -> flow merge/1
  Sum/1 -> TH0011_thermalMass/1
  bypass valve/1 -> TH0011_coolingChannel/2
  TH0011_coolingChannel/1 -> Gain3/1
  TH0011_thermalMass/1 -> T_ [K]/1, TH0011_coolingChannel/1
  bypass valve/2 -> flow merge/2
  valve [-]/1 -> bypass valve/1
  clt_1 (T,p,W)/1 -> bypass valve/2
  flow merge/2 -> bypass valve/3
  Gain3/1 -> Sum/2
  Q_in [J/s]/1 -> Sum/1
